simulink model "h2f_175_plant_model"  (R2023a)
settings: Solver=FixedStepAuto  StartTime=0.0  StopTime=10.0  FixedStep=0.02  RelTol=1e-3
PreLoadFcn:
  | addpath(fullfile('h175_model','thermal'))
  | run('thermal_variants_config.m')
undefined symbols (not defined in the file): b_AmbientSens, b_AnodeSens, b_ARP1_SENS, b_ARP2_SENS, b_auxTCP_SENS, b_CathodeSens, b_CBV_SENS, b_CHUBVd_SENS, b_CHUBVw_SENS, b_CHXV_SENS, b_CSens_H2Amb1, b_CSens_H2Amb2, b_CSIV_SENS, b_CSOV_SENS, b_EAC_SENS, b_EATBV_SENS, b_ECoolingSens, b_ElectricalSens, b_ETCP_SENS, b_ETV_SENS, b_ISens_BoP, b_mdotSens_EACi, b_pSens_Ambt, b_pSens_APRVi, b_pSens_ASti, b_pSens_CLSti, b_pSens_ECL, b_RSens_ISOMON, b_Sens_IVT, b_StackRelay_SENS, b_TCP_SENS, b_TCV_SENS, b_ThermalSens, b_TimeSync, b_TSens_Ambt, b_TSens_ASVi, b_TSens_CLSti, b_TSens_CLSto, b_TSens_CSti, b_TSens_TCVi, b_USens_StCV, clean_data_ThermalSim, gaussian, RELAY_STATE, s_I_A_BOP_Get, s_I_A_StN_Get, s_omega_rpm_ARP1_Get, s_omega_rpm_ARP2_Get, s_omega_rpm_auxTCP_Get, s_omega_rpm_EAC_Get, s_omega_rpm_TCP_Get, s_p_bara_APRVi_Get, s_p_bara_ASti_Get, s_p_bara_CLSti_Get, s_p_bara_CLSto_Sim, s_p_bara_ECL_Get, s_P_W_St_Get, s_pos_enum_StNR_Get, s_pos_enum_StPR_Get, s_pos_per_TCV_Get ... (+92)
libraries: simulink x25, nesl_utility x1
(part 2 of 2)

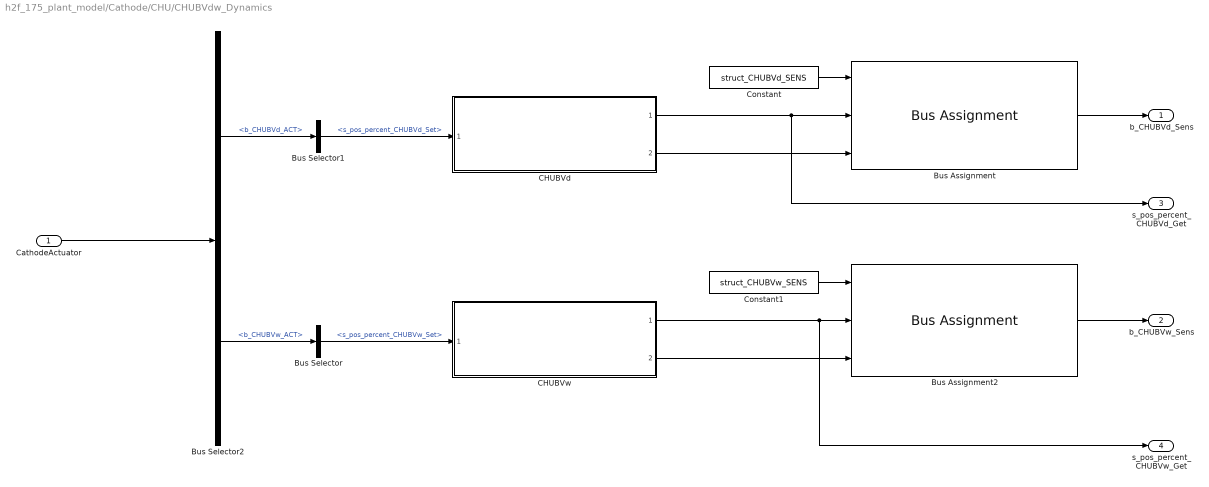
== system h2f_175_plant_model/Cathode/CHU/CHUBVdw_Dynamics ==
  CathodeActuator : Inport  OutDataTypeStr=Bus: CathodeAct
  Bus Assignment : BusAssignment  AssignedSignals=s_pos_percent_CHUBVd_Get,s_st_enum_CHUBVd_Get
  Bus Assignment2 : BusAssignment  AssignedSignals=s_pos_percent_CHUBVw_ACT_Get,s_st_enum_CHUBVw_Get
  Bus Selector : BusSelector  OutputSignals=s_pos_percent_CHUBVw_Set
  Bus Selector1 : BusSelector  OutputSignals=s_pos_percent_CHUBVd_Set
  Bus Selector2 : BusSelector  OutputSignals=b_CHUBVd_ACT,b_CHUBVw_ACT
  CHUBVd : Subsystem  ReferencedSubsystem=OES_Valve
  CHUBVw : Subsystem  ReferencedSubsystem=OES_Valve
  Constant : Constant  Value=struct_CHUBVd_SENS  OutDataTypeStr=Bus: CHUBVd_SENS
  Constant1 : Constant  Value=struct_CHUBVw_SENS  OutDataTypeStr=Bus: CHUBVw_SENS
  b_CHUBVd_Sens : Outport  OutDataTypeStr=Bus: CHUBVd_SENS
  b_CHUBVw_Sens : Outport  Port=2  OutDataTypeStr=Bus: CHUBVw_SENS
  s_pos_percent_CHUBVd_Get : Outport  Port=3  OutDataTypeStr=single
  s_pos_percent_CHUBVw_Get : Outport  Port=4  OutDataTypeStr=single
  wires:
  CHUBVd/2 -> Bus Assignment/3
  Bus Selector1/1 -> CHUBVd/1  "<s_pos_percent_CHUBVd_Set>"
  CHUBVd/1 -> Bus Assignment/2, s_pos_percent_CHUBVd_Get/1
  CHUBVw/1 -> Bus Assignment2/2, s_pos_percent_CHUBVw_Get/1
  Bus Selector2/2 -> Bus Selector/1  "<b_CHUBVw_ACT>"
  Bus Selector2/1 -> Bus Selector1/1  "<b_CHUBVd_ACT>"
  CathodeActuator/1 -> Bus Selector2/1
  Bus Selector/1 -> CHUBVw/1  "<s_pos_percent_CHUBVw_Set>"
  CHUBVw/2 -> Bus Assignment2/3
  Constant1/1 -> Bus Assignment2/1
  Bus Assignment/1 -> b_CHUBVd_Sens/1
  Bus Assignment2/1 -> b_CHUBVw_Sens/1
  Constant/1 -> Bus Assignment/1

== system h2f_175_plant_model/Cathode/CHU/HumidifierDynamics ==
  s_pos_percent_CHUBVd_Get : Inport
  s_pos_percent_CHUBVw_Get : Inport  Port=2
  Ground : Ground
  Terminator : Terminator
  Terminator1 : Terminator
  e.g. Humidity : Outport
  wires:
  s_pos_percent_CHUBVw_Get/1 -> Terminator1/1
  s_pos_percent_CHUBVd_Get/1 -> Terminator/1
  Ground/1 -> e.g. Humidity/1

== system h2f_175_plant_model/Subsystem1/Subsystem4/HVRelays ==
  ElectricalAct : Inport  OutDataTypeStr=Bus: ElectricalAct
  Bus Selector : BusSelector  OutputSignals=b_HVRelays.s_pos_enum_HVPrePR_Set,b_HVRelays.s_pos_enum_HVPR_Set
  Cast To Single : DataTypeConversion  OutDataTypeStr=single  SaturateOnIntegerOverflow=off  RndMeth=Floor
  Constant1 : Constant  Value=0
  Constant2 : Constant  Value=450
  Enumerated Constant : simulink/Sources/Enumerated Constant  OutDataTypeStr=Enum: RELAY_STATE  Value=RELAY_STATE.Connected  SampleTime=inf
  Equal : RelationalOperator  Operator===  OutDataTypeStr=boolean  RndMeth=Simplest  InputSameDT=off
  Equal1 : RelationalOperator  Operator===  OutDataTypeStr=boolean  RndMeth=Simplest  InputSameDT=off
  OR : Logic  Operator=OR  IconShape=distinctive  AllPortsSameDT=off  OutDataTypeStr=boolean
  Switch : Switch  Criteria=u2 > Threshold  SaturateOnIntegerOverflow=off  InputSameDT=off
  HighVoltage_V : Outport
  wires:
  ElectricalAct/1 -> Bus Selector/1
  Bus Selector/1 -> Equal/2  "<s_pos_enum_HVPrePR_Set>"
  Constant1/1 -> Switch/3
  Constant2/1 -> Switch/1
  Switch/1 -> Cast To Single/1
  Bus Selector/2 -> Equal1/2  "<s_pos_enum_HVPR_Set>"
  Enumerated Constant/1 -> Equal1/1, Equal/1
  Equal/1 -> OR/1
  OR/1 -> Switch/2
  Equal1/1 -> OR/2
  Cast To Single/1 -> HighVoltage_V/1

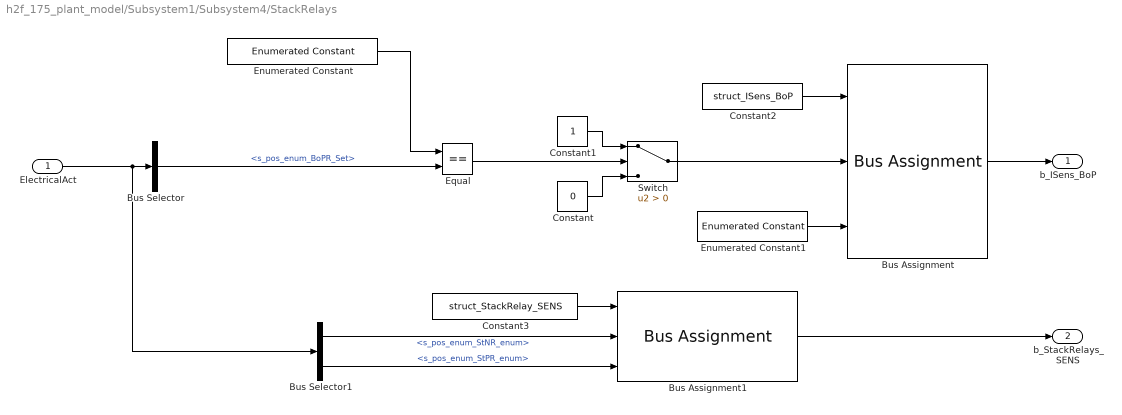
== system h2f_175_plant_model/Subsystem1/Subsystem4/StackRelays ==
  ElectricalAct : Inport  OutDataTypeStr=Bus: ElectricalAct
  Bus Assignment : BusAssignment  AssignedSignals=s_I_A_BOP_Get,s_st_enum_BoP_Get
  Bus Assignment1 : BusAssignment  AssignedSignals=s_pos_enum_StNR_Get,s_pos_enum_StPR_Get
  Bus Selector : BusSelector  OutputSignals=b_BoPRelays.s_pos_enum_BoPR_Set
  Bus Selector1 : BusSelector  OutputSignals=b_StackRelays.s_pos_enum_StNR_enum,b_StackRelays.s_pos_enum_StPR_enum
  Constant : Constant  Value=0  OutDataTypeStr=single
  Constant1 : Constant  OutDataTypeStr=single
  Constant2 : Constant  Value=struct_ISens_BoP  OutDataTypeStr=Bus: ISens_BoP
  Constant3 : Constant  Value=struct_StackRelay_SENS  OutDataTypeStr=Bus: StackRelay_SENS
  Enumerated Constant : simulink/Sources/Enumerated Constant  OutDataTypeStr=Enum: RELAY_STATE  Value=RELAY_STATE.Connected  SampleTime=inf
  Enumerated Constant1 : simulink/Sources/Enumerated Constant  OutDataTypeStr=Enum: SENS_STATUS  Value=SENS_STATUS.OK  SampleTime=inf
  Equal : RelationalOperator  Operator===  OutDataTypeStr=boolean  RndMeth=Simplest  InputSameDT=off
  Switch : Switch  Criteria=u2 > Threshold  SaturateOnIntegerOverflow=off  InputSameDT=off
  b_ISens_BoP : Outport  OutDataTypeStr=Bus: ISens_BoP
  b_StackRelays_SENS : Outport  Port=2  OutDataTypeStr=Bus: StackRelay_SENS
  wires:
  Bus Selector/1 -> Equal/2  "<s_pos_enum_BoPR_Set>"
  Enumerated Constant/1 -> Equal/1
  Equal/1 -> Switch/2
  Constant/1 -> Switch/3
  Constant1/1 -> Switch/1
  Constant2/1 -> Bus Assignment/1
  Switch/1 -> Bus Assignment/2
  Bus Assignment/1 -> b_ISens_BoP/1
  Enumerated Constant1/1 -> Bus Assignment/3
  Bus Assignment1/1 -> b_StackRelays_SENS/1
  Bus Selector1/2 -> Bus Assignment1/3  "<s_pos_enum_StPR_enum>"
  Bus Selector1/1 -> Bus Assignment1/2  "<s_pos_enum_StNR_enum>"
  Constant3/1 -> Bus Assignment1/1
  ElectricalAct/1 -> Bus Selector/1, Bus Selector1/1

== system h2f_175_plant_model/Thermal/Bus Assignment/TCV_Direction_Opening ==
  pos_TCV_per_Set : Inport
  Open_Leads_To_Cooling : Subsystem  TreatAsAtomicUnit=on  VariantControl=variantConfig.TCVDirection == VARIANT_TCVDirection.OPEN_IS_COOLING
  Open_Leads_To_Heating : Subsystem  TreatAsAtomicUnit=on  VariantControl=variantConfig.TCVDirection == VARIANT_TCVDirection.OPEN_IS_HEATING
  pos_TCV_per_Set_out : Outport

== system h2f_175_plant_model/Thermal/TCV_Direction_Opening/Open_Leads_To_Cooling ==
  pos_TCV_per_Set : Inport
  pos_TCV_per_Set_out : Outport
  wires:
  pos_TCV_per_Set/1 -> pos_TCV_per_Set_out/1

== system h2f_175_plant_model/Thermal/TCV_Direction_Opening/Open_Leads_To_Heating ==
  pos_TCV_per_Set : Inport
  Add : Sum  Inputs=+-
  Constant : Constant  Value=100  OutDataTypeStr=single
  pos_TCV_per_Set_out : Outport
  wires:
  Constant/1 -> Add/1
  pos_TCV_per_Set/1 -> Add/2
  Add/1 -> pos_TCV_per_Set_out/1

== system h2f_175_plant_model/Thermal/Bus Assignment/TCV_Direction_Opening/Open_Leads_To_Cooling ==
  pos_TCV_per_Set : Inport
  pos_TCV_per_Set_out : Outport
  wires:
  pos_TCV_per_Set/1 -> pos_TCV_per_Set_out/1

== system h2f_175_plant_model/Thermal/Bus Assignment/TCV_Direction_Opening/Open_Leads_To_Heating ==
  pos_TCV_per_Set : Inport
  Add : Sum  Inputs=+-
  Constant : Constant  Value=100  OutDataTypeStr=single
  pos_TCV_per_Set_out : Outport
  wires:
  Constant/1 -> Add/1
  pos_TCV_per_Set/1 -> Add/2
  Add/1 -> pos_TCV_per_Set_out/1
